simulink model "sampleModel1871_5_sub_sub"  (R2023a)
settings: Solver=VariableStepAuto  StartTime=0.0  StopTime=10.0  RelTol=1e-3
libraries: hdlsllib x1
settings Model: Creator=user1  LastModifiedBy=user1
settings OptimizationCC: BlockReduction=off  ConditionallyExecuteInputs=off

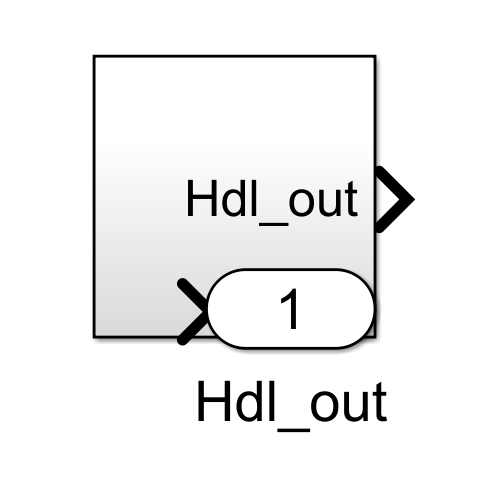
[thumbnail: Simulink's stored preview of the top-level diagram]
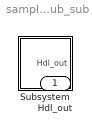
== system sampleModel1871_5_sub_sub ==
  Subsystem : Subsystem
  Hdl_out : Outport  OutDataTypeStr=uint8

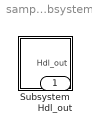
== system sampleModel1871_5_sub_sub/Subsystem ==
  Subsystem : Subsystem
  Hdl_out : Outport  OutDataTypeStr=uint8

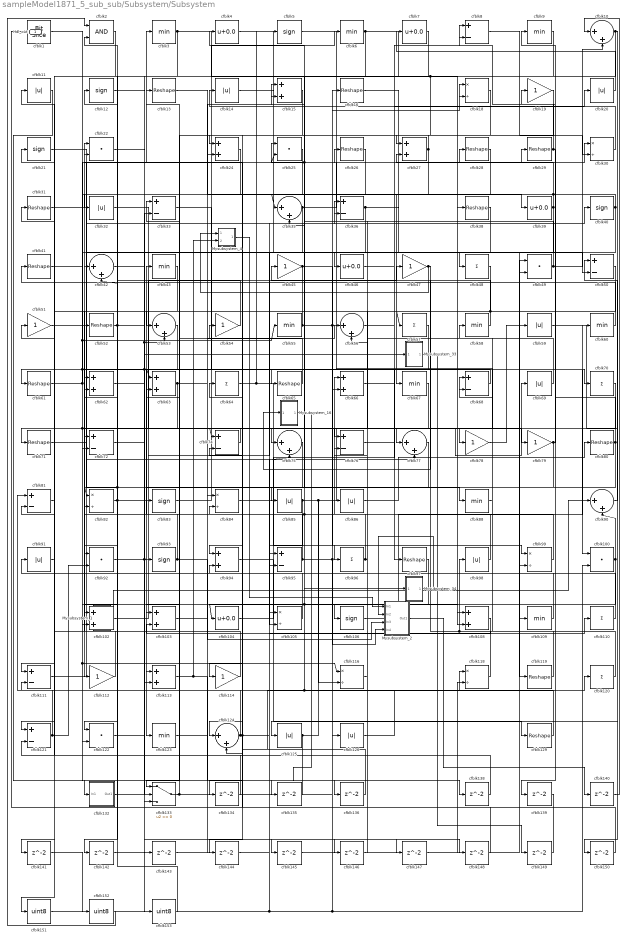
== system sampleModel1871_5_sub_sub/Subsystem/Subsystem ==
  Mysubsystem_1 : Subsystem  TreatAsAtomicUnit=on  RTWFcnName=Mysubsystem_1
      settings: RTWFcnNameOpts=User specified  RTWFileNameOpts=Use function name
  Mysubsystem_16 : Subsystem  TreatAsAtomicUnit=on  RTWFcnName=Mysubsystem_16
      settings: RTWFcnNameOpts=User specified  RTWFileNameOpts=Use function name
  Mysubsystem_2 : Subsystem  TreatAsAtomicUnit=on  RTWFcnName=Mysubsystem_2
      settings: RTWFcnNameOpts=User specified  RTWFileNameOpts=Use function name
  Mysubsystem_33 : Subsystem  TreatAsAtomicUnit=on  RTWFcnName=Mysubsystem_33
      settings: RTWFcnNameOpts=User specified  RTWFileNameOpts=Use function name
  Mysubsystem_34 : Subsystem  TreatAsAtomicUnit=on  RTWFcnName=Mysubsystem_34
      settings: RTWFcnNameOpts=User specified  RTWFileNameOpts=Use function name
  Mysubsystem_4 : Subsystem  TreatAsAtomicUnit=on  RTWFcnName=Mysubsystem_4
      settings: RTWFcnNameOpts=User specified  RTWFileNameOpts=Use function name
  cfblk1 : hdlsllib/Logic and Bit Operations/Bit Slice  lidx=7  ridx=0
  cfblk{10,35,42,53,56,75,77,90,124} (9 alike) : Sum  Inputs=|++  OutDataTypeStr=uint8
  cfblk{22,25,49,92,100,122} (6 alike) : DotProduct  OutDataTypeStr=uint8
  cfblk{15,24,27,62..63,66,94,102..103,108,113} (11 alike) : Sum  OutDataTypeStr=uint8
  cfblk{4,7,39,46,104} (5 alike) : Bias  Bias=0.0  SaturateOnIntegerOverflow=off
  cfblk{18,30,82,84,99,105,116,118} (8 alike) : Product  Inputs=*/  OutDataTypeStr=uint8  RndMeth=Zero  SaturateOnIntegerOverflow=on
  cfblk{5,12,21,40,83,93,106} (7 alike) : Signum
  cfblk{3,6,9,43,55,58,60,67,88,109,123} (11 alike) : MinMax  OutDataTypeStr=uint8
  cfblk{11,14,20,32,59,69,85..86,91,98,125..126} (12 alike) : Abs  OutDataTypeStr=uint8  SaturateOnIntegerOverflow=off
  cfblk{48,57,64,70,96,110,120} (7 alike) : Sum  Inputs=+  OutDataTypeStr=uint8
  cfblk{8,33,36,50,68,72,74,76,81,95,111,121} (12 alike) : Sum  Inputs=+-  OutDataTypeStr=uint8
  cfblk{19,45,47,51,54,78..79,112,114} (9 alike) : Gain  OutDataTypeStr=uint8
  cfblk{13,16,26,28..29,31,38,41,52,61,65,71,80,97,119,129} (16 alike) : Reshape
  cfblk132 : Subsystem
      settings: LibrarySourceBlock=|
      | hdlsllib/Ports &
      | Subsystems/Subsystem
  cfblk133 : Switch  OutDataTypeStr=uint8  SaturateOnIntegerOverflow=off  InputSameDT=off
  cfblk{134..136,138..150} (16 alike) : Delay  SampleTime=1
  cfblk151 : DataTypeConversion  OutDataTypeStr=uint8  SaturateOnIntegerOverflow=off  RndMeth=Floor
  cfblk152 : DataTypeConversion  OutDataTypeStr=uint8  SaturateOnIntegerOverflow=off  RndMeth=Floor
  cfblk153 : DataTypeConversion  OutDataTypeStr=uint8  SaturateOnIntegerOverflow=off  RndMeth=Floor
  cfblk2 : Logic  AllPortsSameDT=off  OutDataTypeStr=boolean
  Hdl_out : Outport  OutDataTypeStr=uint8
  wires:
  Mysubsystem_34/1(Out1) -> Mysubsystem_2/2(In2)
  Mysubsystem_33/1(Out1) -> cfblk149/1
  Mysubsystem_16/1(Out1) -> cfblk138/1
  Mysubsystem_4/1(Out1) -> Mysubsystem_2/1(In1)
  Mysubsystem_2/1(Out1) -> cfblk140/1
  Mysubsystem_1/1(Out1) -> cfblk90/1
  cfblk153/1 -> cfblk2/2
  cfblk62/1 -> cfblk153/1
  cfblk152/1 -> cfblk2/1
  cfblk141/1 -> cfblk152/1
  cfblk151/1 -> cfblk100/2, cfblk126/1, cfblk75/2
  cfblk150/1 -> cfblk74/2
  cfblk149/1 -> cfblk94/2
  cfblk148/1 -> cfblk62/2
  cfblk147/1 -> cfblk118/2
  cfblk146/1 -> cfblk76/2
  cfblk92/1 -> cfblk146/1
  cfblk145/1 -> cfblk49/1
  cfblk72/1 -> cfblk145/1
  cfblk144/1 -> cfblk105/1
  cfblk143/1 -> cfblk84/1
  cfblk42/1 -> cfblk143/1
  cfblk142/1 -> cfblk95/1
  cfblk50/1 -> cfblk141/1
  cfblk140/1 -> cfblk10/1
  cfblk139/1 -> cfblk1/1
  cfblk138/1 -> cfblk121/2
  cfblk136/1 -> cfblk22/2
  cfblk135/1 -> cfblk111/2
  cfblk134/1 -> cfblk81/2
  cfblk18/1 -> cfblk134/1
  cfblk91/1 -> cfblk21/1
  cfblk31/1 -> cfblk48/1
  cfblk47/1 -> Mysubsystem_16/1(In1), Mysubsystem_4/1(In1)
  cfblk24/1 -> cfblk113/2
  cfblk120/1 -> cfblk68/2
  cfblk15/1 -> cfblk24/2
  cfblk12/1 -> cfblk66/2, cfblk148/1
  cfblk39/1 -> cfblk35/1, cfblk27/2, cfblk95/2
  cfblk45/1 -> cfblk102/1, cfblk99/2
  cfblk129/1 -> cfblk11/1, cfblk15/2
  cfblk40/1 -> cfblk49/2, cfblk32/1
  cfblk20/1 -> cfblk7/1
  cfblk74/1 -> cfblk71/1
  cfblk133/1 -> cfblk16/1, cfblk63/2
  cfblk99/1 -> cfblk54/1
  cfblk6/1 -> cfblk108/1, cfblk72/2
  cfblk124/1 -> cfblk110/1, cfblk144/1, cfblk51/1
  cfblk2/1 -> cfblk151/1
  cfblk80/1 -> cfblk19/1, cfblk83/1
  cfblk63/1 -> cfblk72/1, cfblk65/1
  cfblk82/1 -> cfblk36/2, cfblk42/2
  cfblk126/1 -> cfblk118/1
  cfblk94/1 -> cfblk129/1
  cfblk41/1 -> cfblk70/1
  cfblk26/1 -> cfblk122/2
  cfblk116/1 -> cfblk36/1
  cfblk61/1 -> cfblk55/1, cfblk26/1, cfblk63/1, cfblk108/2
  cfblk66/1 -> cfblk18/1
  cfblk96/1 -> cfblk13/1, cfblk25/1, cfblk56/2
  cfblk104/1 -> cfblk29/1
  cfblk3/1 -> cfblk38/1, cfblk133/3
  cfblk52/1 -> cfblk92/1, cfblk82/1, cfblk147/1
  cfblk60/1 -> cfblk41/1
  cfblk108/1 -> cfblk103/2
  cfblk22/1 -> cfblk53/2, cfblk135/1
  cfblk132/1(Out1) -> Mysubsystem_33/1(In1), cfblk93/1
  cfblk71/1 -> cfblk88/1
  cfblk10/1 -> cfblk62/1, cfblk27/1, cfblk150/1
  cfblk95/1 -> Mysubsystem_2/4(In4), cfblk28/1, cfblk82/2
  cfblk19/1 -> cfblk103/1
  cfblk123/1 -> cfblk15/1
  cfblk1/1 -> cfblk116/1, cfblk133/2, cfblk74/1
  cfblk69/1 -> cfblk42/1
  cfblk36/1 -> cfblk50/2, cfblk142/1
  cfblk70/1 -> cfblk113/1
  cfblk122/1 -> cfblk33/2
  cfblk112/1 -> cfblk31/1
  cfblk90/1 -> cfblk50/1
  cfblk88/1 -> cfblk58/1
  cfblk76/1 -> cfblk79/1
  cfblk25/1 -> cfblk124/2
  cfblk84/1 -> cfblk96/1
  cfblk8/1 -> cfblk30/2
  cfblk35/1 -> cfblk30/1, cfblk102/2
  cfblk118/1 -> cfblk98/1, cfblk84/2
  cfblk67/1 -> cfblk122/1
  cfblk81/1 -> cfblk111/1
  cfblk49/1 -> cfblk4/1, cfblk25/2, cfblk10/2
  cfblk93/1 -> Mysubsystem_2/3(In3), cfblk43/1
  cfblk9/1 -> cfblk52/1
  cfblk7/1 -> cfblk75/1
  cfblk100/1 -> cfblk106/1, cfblk90/2
  cfblk4/1 -> cfblk109/1
  cfblk51/1 -> cfblk3/1
  cfblk57/1 -> cfblk121/1
  cfblk29/1 -> cfblk8/2, cfblk139/1
  cfblk43/1 -> cfblk112/1
  cfblk103/1 -> cfblk56/1
  cfblk65/1 -> cfblk33/1
  cfblk64/1 -> cfblk99/1, cfblk5/1
  cfblk38/1 -> cfblk94/1
  cfblk113/1 -> Mysubsystem_4/2(In2), cfblk136/1
  cfblk21/1 -> cfblk77/2
  cfblk75/1 -> cfblk114/1
  cfblk79/1 -> cfblk9/1, cfblk133/1
  cfblk32/1 -> cfblk77/1
  cfblk48/1 -> cfblk76/1
  cfblk56/1 -> cfblk8/1
  cfblk125/1 -> cfblk120/1, cfblk86/1
  cfblk110/1 -> cfblk68/1
  cfblk111/1 -> cfblk40/1
  cfblk97/1 -> Mysubsystem_34/1(In1), cfblk104/1
  cfblk55/1 -> cfblk100/1, cfblk18/2, cfblk53/1
  cfblk33/1 -> cfblk97/1
  cfblk58/1 -> cfblk57/1, cfblk35/2
  cfblk14/1 -> cfblk46/1
  cfblk11/1 -> cfblk132/1(In1)
  cfblk119/1 -> cfblk45/1
  cfblk98/1 -> cfblk66/1
  cfblk27/1 -> cfblk24/1, cfblk85/1
  cfblk16/1 -> cfblk119/1
  cfblk106/1 -> cfblk60/1
  cfblk53/1 -> cfblk123/1
  cfblk46/1 -> cfblk20/1
  cfblk13/1 -> cfblk39/1
  cfblk102/1 -> cfblk47/1
  cfblk30/1 -> cfblk14/1
  cfblk109/1 -> cfblk64/1
  cfblk77/1 -> cfblk124/1
  cfblk59/1 -> cfblk125/1
  cfblk83/1 -> cfblk6/1
  cfblk78/1 -> cfblk59/1
  cfblk54/1 -> cfblk12/1
  cfblk85/1 -> cfblk69/1, cfblk116/2, cfblk105/2
  cfblk121/1 -> cfblk81/1, cfblk92/2
  cfblk105/1 -> cfblk91/1
  cfblk28/1 -> cfblk67/1
  cfblk5/1 -> cfblk78/1
  cfblk68/1 -> cfblk61/1
  cfblk86/1 -> cfblk80/1
  cfblk114/1 -> cfblk22/1

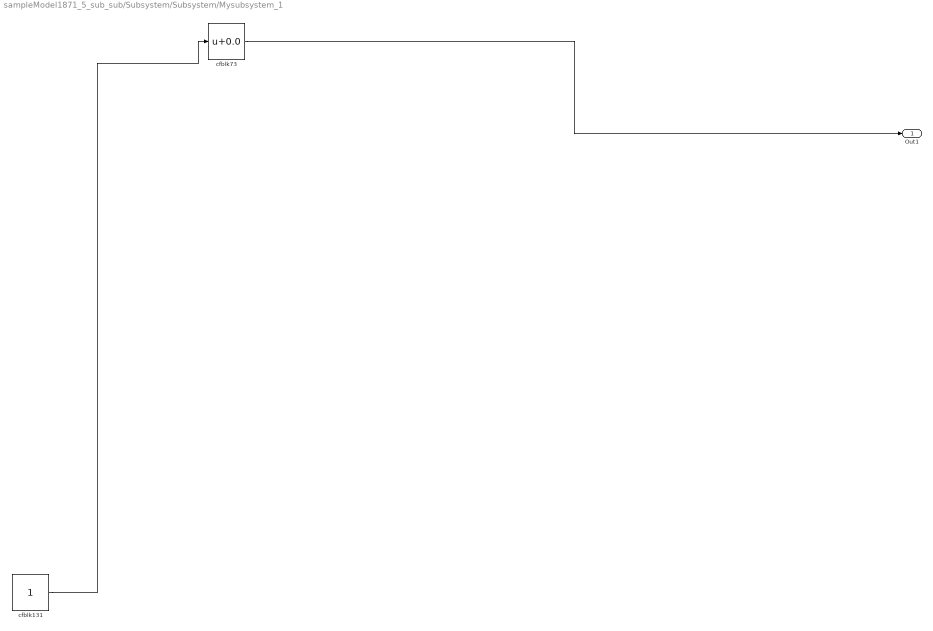
== system sampleModel1871_5_sub_sub/Subsystem/Subsystem/Mysubsystem_1 ==
  cfblk131 : Constant  SampleTime=-1
  cfblk73 : Bias  Bias=0.0  SaturateOnIntegerOverflow=off
  Out1 : Outport
  wires:
  cfblk131/1 -> cfblk73/1
  cfblk73/1 -> Out1/1

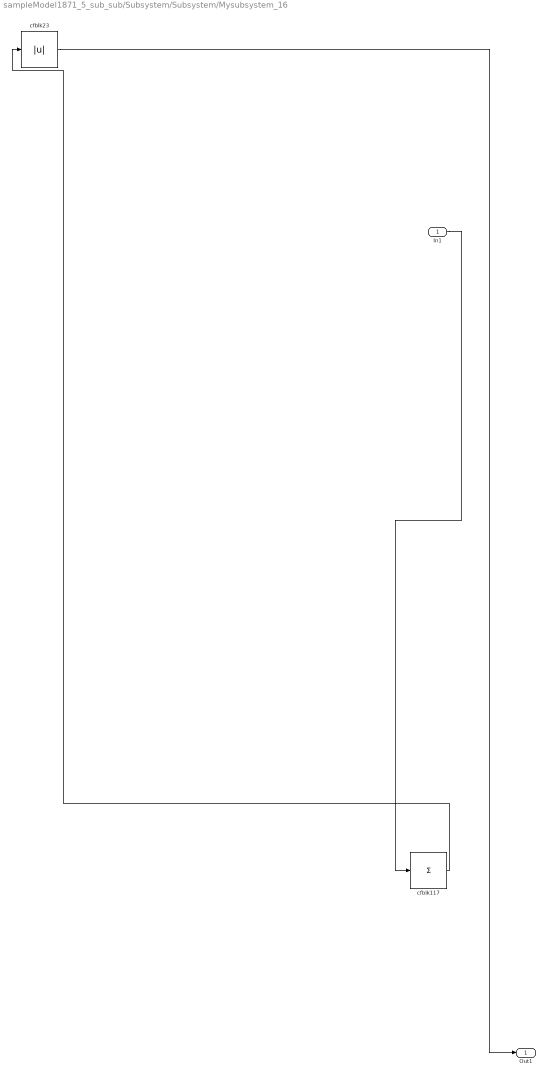
== system sampleModel1871_5_sub_sub/Subsystem/Subsystem/Mysubsystem_16 ==
  In1 : Inport
  cfblk117 : Sum  Inputs=+
  cfblk23 : Abs  SaturateOnIntegerOverflow=off
  Out1 : Outport
  wires:
  cfblk117/1 -> cfblk23/1
  In1/1 -> cfblk117/1
  cfblk23/1 -> Out1/1

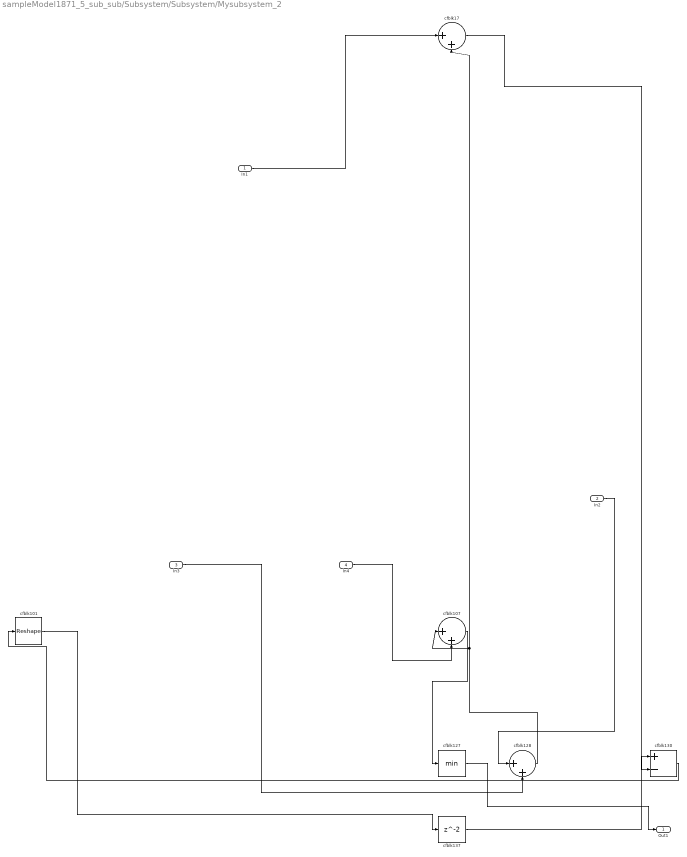
== system sampleModel1871_5_sub_sub/Subsystem/Subsystem/Mysubsystem_2 ==
  In1 : Inport
  In2 : Inport  Port=2
  In3 : Inport  Port=3
  In4 : Inport  Port=4
  cfblk101 : Reshape
  cfblk107 : Sum  Inputs=|++
  cfblk127 : MinMax
  cfblk128 : Sum  Inputs=|++
  cfblk130 : Sum  Inputs=+-
  cfblk137 : Delay  SampleTime=1
  cfblk17 : Sum  Inputs=|++
  Out1 : Outport
  wires:
  cfblk128/1 -> cfblk17/2, cfblk107/1
  cfblk101/1 -> cfblk137/1
  cfblk107/1 -> cfblk127/1
  cfblk130/1 -> cfblk101/1
  cfblk17/1 -> cfblk130/2
  cfblk137/1 -> cfblk130/1
  cfblk127/1 -> Out1/1
  In2/1 -> cfblk128/1
  In3/1 -> cfblk128/2
  In1/1 -> cfblk17/1
  In4/1 -> cfblk107/2

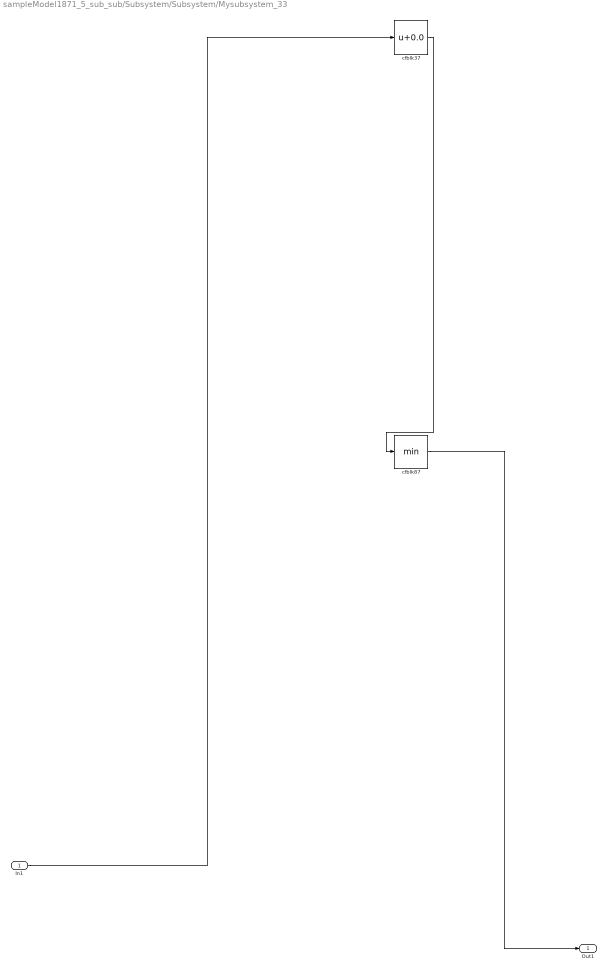
== system sampleModel1871_5_sub_sub/Subsystem/Subsystem/Mysubsystem_33 ==
  In1 : Inport
  cfblk37 : Bias  Bias=0.0  SaturateOnIntegerOverflow=off
  cfblk87 : MinMax
  Out1 : Outport
  wires:
  cfblk37/1 -> cfblk87/1
  cfblk87/1 -> Out1/1
  In1/1 -> cfblk37/1

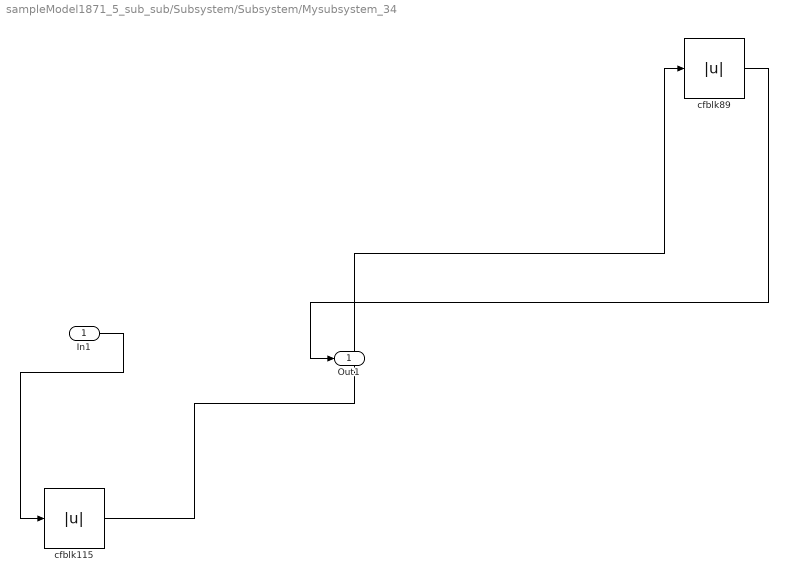
== system sampleModel1871_5_sub_sub/Subsystem/Subsystem/Mysubsystem_34 ==
  In1 : Inport
  cfblk115 : Abs  SaturateOnIntegerOverflow=off
  cfblk89 : Abs  SaturateOnIntegerOverflow=off
  Out1 : Outport
  wires:
  cfblk115/1 -> cfblk89/1
  cfblk89/1 -> Out1/1
  In1/1 -> cfblk115/1

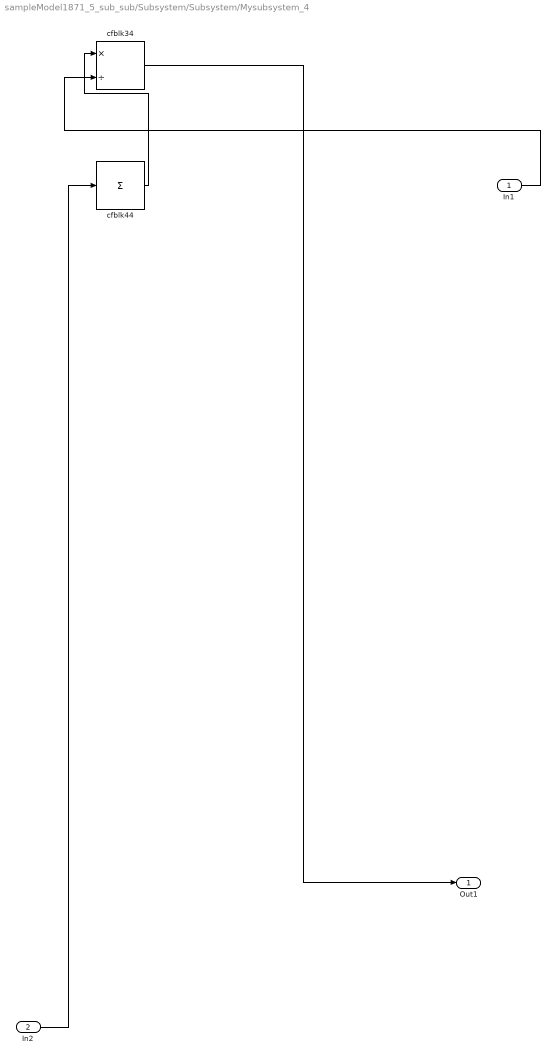
== system sampleModel1871_5_sub_sub/Subsystem/Subsystem/Mysubsystem_4 ==
  In1 : Inport
  In2 : Inport  Port=2
  cfblk34 : Product  Inputs=*/  RndMeth=Zero  SaturateOnIntegerOverflow=on
  cfblk44 : Sum  Inputs=+
  Out1 : Outport
  wires:
  In1/1 -> cfblk34/2
  cfblk44/1 -> cfblk34/1
  In2/1 -> cfblk44/1
  cfblk34/1 -> Out1/1

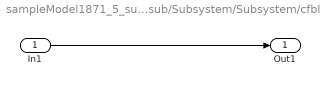
== system sampleModel1871_5_sub_sub/Subsystem/Subsystem/cfblk132 ==
  In1 : Inport
  Out1 : Outport
  wires:
  In1/1 -> Out1/1
